simulink model "sl_braitenberg"  (Simulink 7.9)
settings: Solver=ode45  StartTime=0.0  StopTime=200  RelTol=1e-3
undefined symbols (not defined in the file or in its folder): se2
libraries: roblocks x1, simulink x1
settings Model: Creator=pic  LastModifiedBy=corkep
settings DataIOCC: SaveOutput=off  SaveState=on
settings DebuggingCC: FcnCallInpInsideContextMsg=Use local settings  StrictBusMsg=Warning
settings GRTTargetCC: CombineOutputUpdateFcns=off  GRTInterface=on

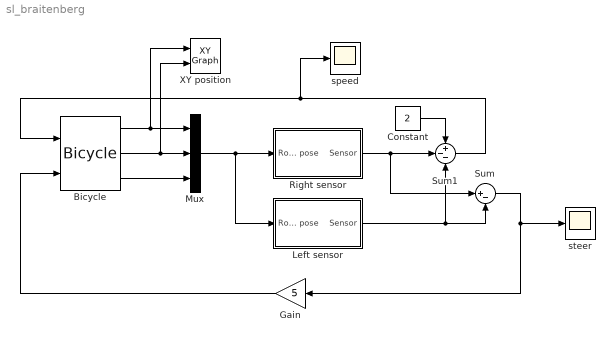
== system sl_braitenberg ==
  Bicycle : roblocks/Dynamics/Bicycle  accel=1  vlim=1  alim=2  L=1  x0=[5, 5, 0]  handbrake=0
  Constant : Constant  Value=2
  Gain : Gain  Gain=5
  Left sensor : Subsystem  mask{dx=0, dy=-2, sensorfunc=@sensorfield}
      mask prompts: dx "Sensor position x"; dy "Sensor position y"; sensorfunc "Sensor function"
  Mux : Mux  Inputs=3
  Right sensor : Subsystem  mask{dx=0, dy=2, sensorfunc=@sensorfield}
      mask prompts: dx "Sensor position x"; dy "Sensor position y"; sensorfunc "Sensor function"
  Sum : Sum  Inputs=|+-
  Sum1 : Sum  Inputs=+--
  XY position : simulink/Sinks/XY Graph  xmin=0  xmax=100  ymin=0  ymax=100  st=-1
  speed : Scope
      settings: YMin=0.035  YMax=0.0675
  steer : Scope
      settings: YMin=0.035  YMax=0.0675
  wires:
  Bicycle/1 -> Mux/1, XY position/1
  Bicycle/2 -> Mux/2, XY position/2
  Bicycle/3 -> Mux/3
  Mux/1 -> Right sensor/1(Robot pose), Left sensor/1(Robot pose)
  Sum/1 -> steer/1, Gain/1
  Right sensor/1(Sensor) -> Sum/1, Sum1/2
  Left sensor/1(Sensor) -> Sum/2, Sum1/3
  Sum1/1 -> Bicycle/1, speed/1
  Constant/1 -> Sum1/1
  Gain/1 -> Bicycle/2

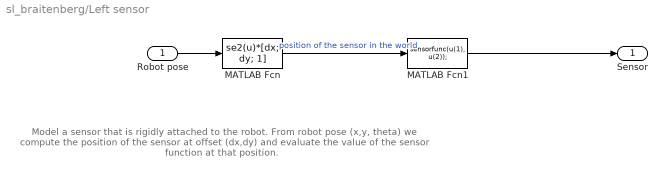
== system sl_braitenberg/Left sensor ==
  note: Model a sensor that is rigidly attached to the robot.
      | From robot pose (x,y, theta) we compute the position of
      | the sensor at offset (dx,dy) and evaluate the value
      | of the sensor function at that position.
  Robot pose : Inport
  MATLAB Fcn : MATLABFcn  MATLABFcn=se2(u)*[dx; dy; 1]
  MATLAB Fcn1 : MATLABFcn  MATLABFcn=sensorfunc(u(1), u(2));  OutputDimensions=1
  Sensor : Outport
  wires:
  Robot pose/1 -> MATLAB Fcn/1
  MATLAB Fcn/1 -> MATLAB Fcn1/1  "position of the sensor in the world"
  MATLAB Fcn1/1 -> Sensor/1

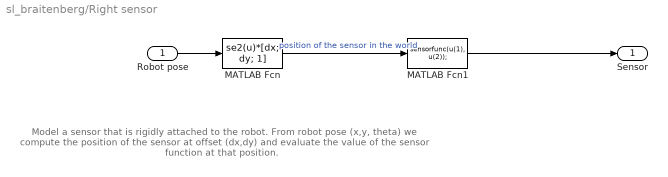
== system sl_braitenberg/Right sensor ==
  note: Model a sensor that is rigidly attached to the robot.
      | From robot pose (x,y, theta) we compute the position of
      | the sensor at offset (dx,dy) and evaluate the value
      | of the sensor function at that position.
  Robot pose : Inport
  MATLAB Fcn : MATLABFcn  MATLABFcn=se2(u)*[dx; dy; 1]
  MATLAB Fcn1 : MATLABFcn  MATLABFcn=sensorfunc(u(1), u(2));  OutputDimensions=1
  Sensor : Outport
  wires:
  Robot pose/1 -> MATLAB Fcn/1
  MATLAB Fcn/1 -> MATLAB Fcn1/1  "position of the sensor in the world"
  MATLAB Fcn1/1 -> Sensor/1
